simulink model "vx_vy_feedback_track_v2_4d_runtime"  (R2024a)
settings: Solver=FixedStepDiscrete  StartTime=0  StopTime=0.1  FixedStep=0.01  RelTol=1e-3
libraries: simulink x1
Description:
  | V2.4-C STANDALONE F-TRACK. P0_F=0.5 and Q_F=0.0025 are TEST-ONLY / UNTUNED / UNFROZEN integration values.
settings Model: Creator=21180  LastModifiedBy=21180

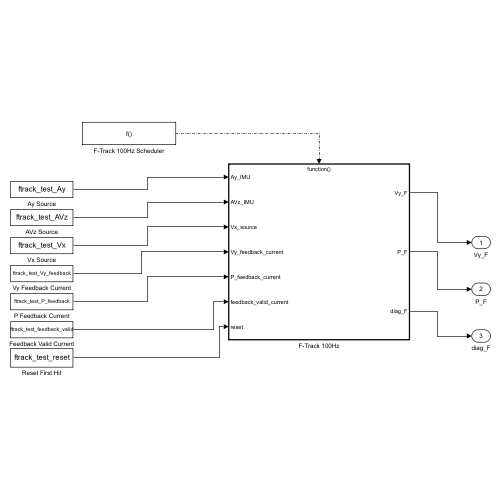
[thumbnail: Simulink's stored preview of the top-level diagram]
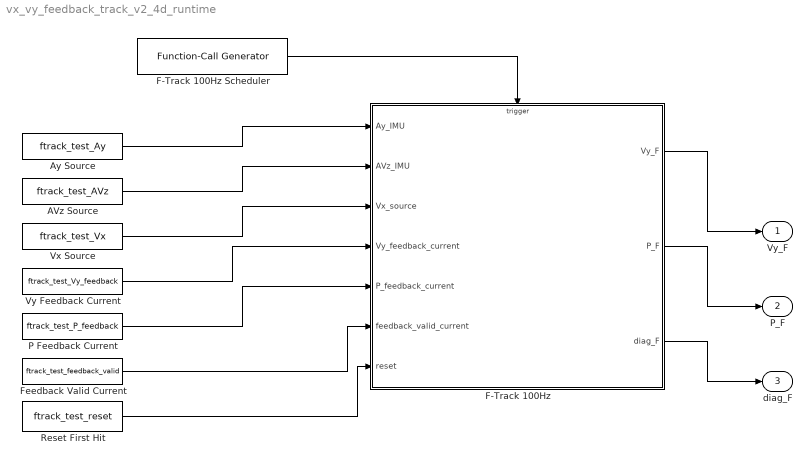
== system vx_vy_feedback_track_v2_4d_runtime ==
  AVz Source : FromWorkspace  VariableName=ftrack_test_AVz  SampleTime=0.01  Interpolate=off  OutputAfterFinalValue=Holding final value
  Ay Source : FromWorkspace  VariableName=ftrack_test_Ay  SampleTime=0.01  Interpolate=off  OutputAfterFinalValue=Holding final value
  F-Track 100Hz : Subsystem  TreatAsAtomicUnit=on
  F-Track 100Hz Scheduler : simulink/Ports & Subsystems/Function-Call Generator  sample_time=0.01  numberOfIterations=1  DisallowWideOutput=off
  Feedback Valid Current : FromWorkspace  VariableName=ftrack_test_feedback_valid  SampleTime=0.01  Interpolate=off  OutputAfterFinalValue=Holding final value
  P Feedback Current : FromWorkspace  VariableName=ftrack_test_P_feedback  SampleTime=0.01  Interpolate=off  OutputAfterFinalValue=Holding final value
  Reset First Hit : FromWorkspace  VariableName=ftrack_test_reset  SampleTime=0.01  Interpolate=off  OutputAfterFinalValue=Holding final value
  Vx Source : FromWorkspace  VariableName=ftrack_test_Vx  SampleTime=0.01  Interpolate=off  OutputAfterFinalValue=Holding final value
  Vy Feedback Current : FromWorkspace  VariableName=ftrack_test_Vy_feedback  SampleTime=0.01  Interpolate=off  OutputAfterFinalValue=Holding final value
  Vy_F : Outport
  P_F : Outport  Port=2
  diag_F : Outport  Port=3
  wires:
  F-Track 100Hz Scheduler/1 -> F-Track 100Hz/Trigger
  F-Track 100Hz/1(Vy_F) -> Vy_F/1
  F-Track 100Hz/2(P_F) -> P_F/1
  F-Track 100Hz/3(diag_F) -> diag_F/1
  Ay Source/1 -> F-Track 100Hz/1(Ay_IMU)
  AVz Source/1 -> F-Track 100Hz/2(AVz_IMU)
  Vx Source/1 -> F-Track 100Hz/3(Vx_source)
  Vy Feedback Current/1 -> F-Track 100Hz/4(Vy_feedback_current)
  P Feedback Current/1 -> F-Track 100Hz/5(P_feedback_current)
  Feedback Valid Current/1 -> F-Track 100Hz/6(feedback_valid_current)
  Reset First Hit/1 -> F-Track 100Hz/7(reset)

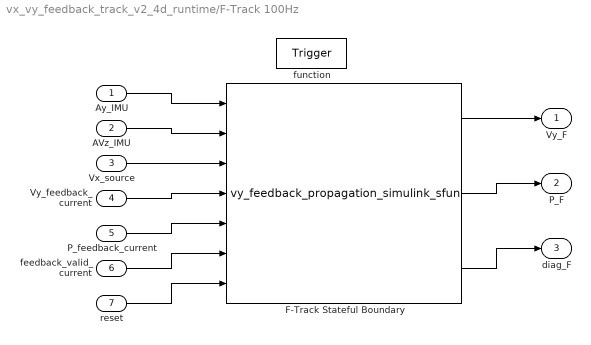
== system vx_vy_feedback_track_v2_4d_runtime/F-Track 100Hz ==
  Ay_IMU : Inport
  AVz_IMU : Inport  Port=2
  Vx_source : Inport  Port=3
  Vy_feedback_current : Inport  Port=4
  P_feedback_current : Inport  Port=5
  feedback_valid_current : Inport  Port=6
  reset : Inport  Port=7
  function : TriggerPort  TriggerType=function-call  VariantControl=(inherit)
  F-Track Stateful Boundary : M-S-Function  FunctionName=vy_feedback_propagation_simulink_sfun  Parameters=0.01,0,0.5,0.0025
  Vy_F : Outport
  P_F : Outport  Port=2
  diag_F : Outport  Port=3
  wires:
  Ay_IMU/1 -> F-Track Stateful Boundary/1
  AVz_IMU/1 -> F-Track Stateful Boundary/2
  Vx_source/1 -> F-Track Stateful Boundary/3
  Vy_feedback_current/1 -> F-Track Stateful Boundary/4
  P_feedback_current/1 -> F-Track Stateful Boundary/5
  feedback_valid_current/1 -> F-Track Stateful Boundary/6
  reset/1 -> F-Track Stateful Boundary/7
  F-Track Stateful Boundary/1 -> Vy_F/1
  F-Track Stateful Boundary/2 -> P_F/1
  F-Track Stateful Boundary/3 -> diag_F/1
